simulink model "adarbha_HW9_sim"  (Simulink 7.7)
settings: Solver=ode1  StartTime=0.0  StopTime=900  FixedStep=0.01  RelTol=1e-2
undefined symbols (not defined in the file): area_sq_m, Cd, density, FUEL_FLOW, OMEGA_ICE, Q, R_batt, radius_wheel_m, rpm, Time, time_s, torque, TORQUE_ICE, V_o, vel_m_s, Velocity_kph, weight_N
libraries: simulink x6
settings Model: Creator=Arjun  LastModifiedBy=Arjun

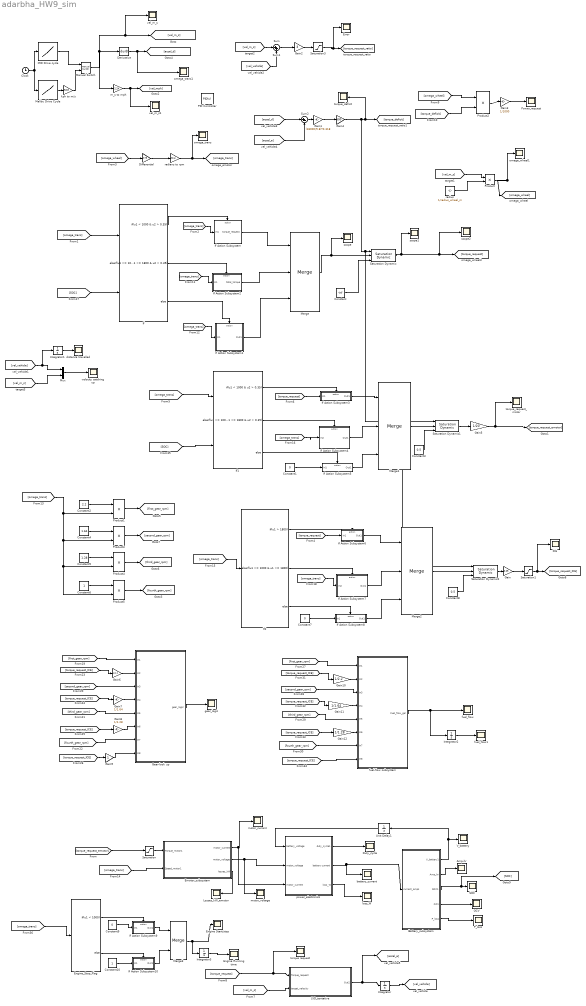
== system adarbha_HW9_sim ==
  Amp-hr : Scope
      settings: SaveName=ScopeData32
  Battery_subsystem : Subsystem
  Clock : Clock
      settings: Decimation=10
  Constant : Constant  Value=-Inf
  Constant1 : Constant  Value=0
  Constant10 : Constant
  Constant2 : Constant  Value=2.2
  Constant3 : Constant  Value=0.5
  Constant4 : Constant  Value=1.64
  Constant5 : Constant  Value=1.28
  Constant6 : Constant
  Constant7 : Constant  Value=0
  Constant8 : Constant  Value=0.5
  Constant9 : Constant  Value=0
  Derivative : Derivative
  Differential : Gain  Gain=3.73
  Duty_cycle : Scope
      settings: SaveName=ScopeData34
  Emotor_subsystem : Subsystem
  Engine Running time : Scope
      settings: SaveName=ScopeData61
  Engine Start/stop : Scope
      settings: SaveName=ScopeData60
  Engine_Stop_Flag : If  IfExpression=u1 < 1000
  Error : Scope
      settings: SaveName=ScopeData17
  Gain : Gain  Gain=0.25
  Gain1 : Gain  Gain=(18000/9.8)*0.318
  Gain10 : Gain  Gain=1/2.2
  Gain11 : Gain  Gain=1/1.64
  Gain12 : Gain  Gain=1/1.28
  Gain2 : Gain  Gain=3
  Gain3 : Gain  Gain=1/1000
  Gain4 : Gain  Gain=500
  Gain5 : Gain  Gain=1/20
  Gain6 : Gain  Gain=1/2.2
  Gain7 : Gain  Gain=1/1.64
  Gain8 : Gain  Gain=1/1.28
  Gain9 : Gain
  Gear-look up : Subsystem
  ICE : Scope
      settings: SaveName=ScopeData44
  If : If  NumInputs=2  IfExpression=u1 < 1000 & u2 > 0.35  ElseIfExpressions=u1 >= 1000 | u1 <= 1800 & u2 > 0.35
  If Action Subsystem : Subsystem  TreatAsAtomicUnit=on
  If Action Subsystem1 : Subsystem  TreatAsAtomicUnit=on
  If Action Subsystem10 : Subsystem  TreatAsAtomicUnit=on
  If Action Subsystem2 : Subsystem  TreatAsAtomicUnit=on
  If Action Subsystem3 : Subsystem  TreatAsAtomicUnit=on
  If Action Subsystem4 : Subsystem  TreatAsAtomicUnit=on
  If Action Subsystem5 : Subsystem  TreatAsAtomicUnit=on
  If Action Subsystem6 : Subsystem  TreatAsAtomicUnit=on
  If Action Subsystem7 : Subsystem  TreatAsAtomicUnit=on
  If Action Subsystem8 : Subsystem  TreatAsAtomicUnit=on
  If Action Subsystem9 : Subsystem  TreatAsAtomicUnit=on
  If1 : If  NumInputs=2  IfExpression=u1 < 1000 & u2 > 0.35  ElseIfExpressions=u1 >= 1000 | u1 <= 1800 & u2 > 0.35
  If2 : If  IfExpression=u1 > 1800  ElseIfExpressions=u1 >= 1000 & u1 <= 1800
  Integrator{,1..3} (4 alike) : Integrator
  LVD_tentative : Subsystem
  Losses_kW_emotor : Scope
      settings: SaveName=ScopeData36
  MID Drive cycle : Lookup_n-D  NumberOfTableDimensions=1  BreakpointsForDimension1=time_s  Table=vel_m_s  RndMeth=Simplest  InputSameDT=on
  Malibu Drive Cycle : Lookup_n-D  NumberOfTableDimensions=1  BreakpointsForDimension1=Time  Table=Velocity_kph  RndMeth=Simplest  InputSameDT=on
  Manual Switch : simulink/Signal Routing/Manual Switch  SystemSampleTime=-1  sw=0  action=0  varsize=off
  Merge : Merge  Inputs=3
  Merge1 : Merge  Inputs=3
  Merge2 : Merge  Inputs=3
  Merge3 : Merge
  Mux : Mux  Inputs=2
  OCV : Scope
      settings: SaveName=ScopeData31
  PID Controller : simulink/Continuous/PID Controller  SystemSampleTime=-1  Controller=PID  TimeDomain=Continuous-time  SampleTime=1  IntegratorMethod=Forward Euler  FilterMethod=Forward Euler  Form=Parallel  P=0.3  I=0  D=0.5  N=100  InitialConditionSource=internal  InitialConditionForIntegrator=0  InitialConditionForFilter=0  ExternalReset=none  LimitOutput=off  UpperSaturationLimit=inf  LowerSaturationLimit=-inf  LinearizeAsGain=off  AntiWindupMode=none  Kb=1  TrackingMode=off  Kt=1  PParamMin=[]  PParamMax=[]  IParamMin=[]  IParamMax=[]  DParamMin=[]  DParamMax=[]  NParamMin=[]  NParamMax=[]  KbParamMin=[]  KbParamMax=[]  KtParamMin=[]  KtParamMax=[]  POutMin=[]  POutMax=[]  IOutMin=[]  IOutMax=[]  DOutMin=[]  DOutMax=[]  NOutMin=[]  NOutMax=[]  KbOutMin=[]  KbOutMax=[]  KtOutMin=[]  KtOutMax=[]  IntegratorOutMin=[]  IntegratorOutMax=[]  FilterOutMin=[]  FilterOutMax=[]  SumOutMin=[]  SumOutMax=[]  SumI1OutMin=[]  SumI1OutMax=[]  SumI2OutMin=[]  SumI2OutMax=[]  SumI3OutMin=[]  SumI3OutMax=[]  SumDOutMin=[]  SumDOutMax=[]  SaturationOutMin=[]  SaturationOutMax=[]  IntegratorContinuousStateAttributes=''  IntegratorStateMustResolveToSignalObject=off  IntegratorRTWStateStorageClass=Auto  FilterContinuousStateAttributes=''  FilterStateMustResolveToSignalObject=off  FilterRTWStateStorageClass=Auto
  P_loss : Scope
      settings: SaveName=ScopeData33
  Power_request : Scope
      settings: SaveName=ScopeData19
  Product{,1..5} (6 alike) : Product  RndMeth=Zero
  SOC : Scope
      settings: SaveName=ScopeData37
  Saturation : Saturate  UpperLimit=100000000  LowerLimit=-2160
  Saturation Dynamic : simulink/Discontinuities/Saturation Dynamic  SystemSampleTime=-1  OutMin=1  OutMax=[]  OutDataTypeStr=Inherit: Same as second input  OutDataType=fixdt(1, 16)  OutScaling=2^-10  DoSatur=off
  Saturation Dynamic1 : simulink/Discontinuities/Saturation Dynamic  SystemSampleTime=-1  OutMin=1  OutMax=[]  OutDataTypeStr=Inherit: Same as second input  OutDataType=fixdt(1, 16)  OutScaling=2^-10  DoSatur=off
  Saturation Dynamic2 : simulink/Discontinuities/Saturation Dynamic  SystemSampleTime=-1  OutMin=1  OutMax=[]  OutDataTypeStr=Inherit: Same as second input  OutDataType=fixdt(1, 16)  OutScaling=2^-10  DoSatur=off
  Saturation1 : Saturate  UpperLimit=10000000  LowerLimit=0
  Saturation3 : Saturate  UpperLimit=1  LowerLimit=-1
  Sum : Sum  Inputs=|+-
  Sum1 : Sum  Inputs=|++
  Sum2 : Sum  Inputs=|+-
  Unit Delay1 : UnitDelay  SampleTime=-1
  V_battery : Scope
      settings: TimeRange=500  YMin=-50  YMax=300  SaveName=ScopeData29
  battery_current : Scope
      settings: SaveName=ScopeData24
  distance travelled : Scope
      settings: SaveName=ScopeData25
  fuel-flow subsystem : Subsystem
  fuel_flow : Scope
      settings: SaveName=ScopeData46
  fuel_flow1 : Scope
      settings: SaveName=ScopeData59
  gear_logic : Scope
      settings: SaveName=ScopeData45
  kph to m/s : Gain  Gain=5/18
  loss_W : Scope
      settings: SaveName=ScopeData38
  m_s to mph : Gain  Gain=2.24
  motor_current : Scope
      settings: SaveName=ScopeData39
  motor_voltage : Scope
      settings: SaveName=ScopeData26
  omega_trans : Scope
      settings: YMin=0  YMax=40  SaveName=ScopeData16
  omega_trans1 : Scope
      settings: YMin=0  YMax=40  SaveName=ScopeData41
  omega_wheel1 : Scope
      settings: SaveName=ScopeData4
  power_electronics : Subsystem
  radians to rpm : Gain  Gain=30/pi
  radius : Constant  Value=1/radius_wheel_m
  scope : Scope
      settings: SaveName=ScopeData3
  scope1 : Scope
      settings: SaveName=ScopeData7
  scope2 : Scope
      settings: SaveName=ScopeData20
  torque request : Scope
      settings: SaveName=ScopeData12
  torque_deficit : Scope
  torque_request_motor : Scope
  vel_m_s : Scope
      settings: TimeRange=49.80784012298233  YMin=0  YMax=30  SaveName=ScopeData21
  vel_m_s1 : Scope
      settings: YMin=0  YMax=40  SaveName=ScopeData28
  velocity catching up : Scope
      settings: TimeRange=765.8724058416602  YMin=-1e+049  YMax=9.000000000000001e+049  SaveName=ScopeData18  SampleTime=800
  wires:
  m_s to mph/1 -> [vel_mph], vel_m_s1/1
  Clock/1 -> MID Drive cycle/1, Malibu Drive Cycle/1
  [vel_m_s] -> Product/1
  Product/1 -> [omega_wheel], omega_wheel1/1
  radius/1 -> Product/2
  [omega_wheel] -> Differential/1
  [vel_m_s] -> LVD_tentative/2(target_velocity)
  [torque_request] -> LVD_tentative/1(Torque_request), torque request/1
  Integrator/1 -> [vel_vehicle]
  LVD_tentative/1(Out2) -> Integrator/1, [accel_a]
  [vel_m_s] -> Sum/1
  [vel_vehicle] -> Sum/2
  [vel_m_s] -> Mux/2
  [vel_vehicle] -> Mux/1, Integrator1/1
  MID Drive cycle/1 -> Manual Switch/1
  Manual Switch/1 -> m_s to mph/1, [vel_m_s], vel_m_s/1, Derivative/1
  Malibu Drive Cycle/1 -> kph to m/s/1
  kph to m/s/1 -> Manual Switch/2
  Integrator1/1 -> distance travelled/1
  Gain2/1 -> Saturation3/1
  Sum/1 -> Gain2/1
  Mux/1 -> velocity catching up/1
  Derivative/1 -> [accel_d], omega_trans1/1
  [accel_d] -> Sum2/1
  [accel_a] -> Sum2/2
  Sum2/1 -> Gain1/1
  Gain1/1 -> Gain4/1
  Saturation3/1 -> [torque_request_ratio], Error/1
  [omega_trans] -> If/1
  If/1 -> If Action Subsystem/Action
  [omega_trans] -> If Action Subsystem/1(In1)
  If/2 -> If Action Subsystem2/Action
  [omega_wheel] -> Product2/1
  [torque_deficit] -> Product2/2
  Product2/1 -> Gain3/1
  Gain3/1 -> Power_request/1
  [omega_trans] -> If Action Subsystem2/1(In1)
  radians to rpm/1 -> [omega_trans], omega_trans/1
  Differential/1 -> radians to rpm/1
  [omega_trans] -> If Action Subsystem1/1(In1)
  If/3 -> If Action Subsystem1/Action
  If Action Subsystem/1(torque_request) -> Merge/1
  If Action Subsystem2/1(total_torque) -> Merge/2
  If Action Subsystem1/1(Out1) -> Merge/3
  Saturation Dynamic/1 -> scope1/1, [torque_request], scope2/1
  Constant/1 -> Saturation Dynamic/3
  Merge/1 -> Saturation Dynamic/2, scope/1
  [omega_trans] -> If1/1
  If1/1 -> If Action Subsystem3/Action
  [torque_request] -> If Action Subsystem3/1(In1)
  If1/2 -> If Action Subsystem4/Action
  If1/3 -> If Action Subsystem5/Action
  Constant1/1 -> If Action Subsystem5/1(In1)
  If Action Subsystem3/1(Out1) -> Merge1/1
  If Action Subsystem4/1(Out1) -> Merge1/2
  If Action Subsystem5/1(Out1) -> Merge1/3
  power_electronics/2(battery current) -> battery_current/1, Battery_subsystem/1(current_amps)
  Battery_subsystem/1(V_battery1) -> V_battery/1, Unit Delay1/1
  Battery_subsystem/3(SOC1) -> SOC/1, [SOC]
  power_electronics/3(loss_W) -> loss_W/1
  power_electronics/1(duty_cycle1) -> Duty_cycle/1
  Battery_subsystem/2(Amp_hr) -> Amp-hr/1
  Battery_subsystem/4(OCV) -> OCV/1
  Battery_subsystem/5(P_loss) -> P_loss/1
  Unit Delay1/1 -> power_electronics/1(battery_voltage)
  Emotor_subsystem/3(losses_kW) -> Losses_kW_emotor/1
  Emotor_subsystem/2(motor_voltage) -> power_electronics/2(motor_voltage), motor_voltage/1
  Emotor_subsystem/1(motor_current) -> motor_current/1, power_electronics/3(motor_current)
  [torque_request_emotor] -> Saturation/1
  [omega_trans] -> Emotor_subsystem/2(Speed_motor1)
  Gain4/1 -> [torque_deficit], torque_deficit/1, Saturation Dynamic/1, Saturation Dynamic1/1, Saturation Dynamic2/1
  [omega_trans] -> If Action Subsystem4/1(In2)
  Merge1/1 -> Saturation Dynamic1/2
  Constant3/1 -> Saturation Dynamic1/3
  Saturation Dynamic1/1 -> Gain5/1
  Saturation/1 -> Emotor_subsystem/1(Torque_motor1)
  [omega_trans] -> Product1/2, Product3/2, Product4/2, Product5/2
  Constant2/1 -> Product1/1
  Constant4/1 -> Product3/1
  Constant5/1 -> Product4/1
  Constant6/1 -> Product5/1
  Product1/1 -> [first_gear_rpm]
  Product3/1 -> [second_gear_rpm]
  Product4/1 -> [third_gear_rpm]
  Product5/1 -> [fourth_gear_rpm]
  [omega_trans] -> If2/1
  If2/1 -> If Action Subsystem6/Action
  If2/2 -> If Action Subsystem7/Action
  [omega_trans] -> If Action Subsystem7/1(In2)
  If2/3 -> If Action Subsystem8/Action
  Constant7/1 -> If Action Subsystem8/1(In1)
  If Action Subsystem8/1(Out1) -> Merge2/3
  If Action Subsystem7/1(Out1) -> Merge2/2
  If Action Subsystem6/1(Out1) -> Merge2/1
  Merge2/1 -> Saturation Dynamic2/2
  Constant8/1 -> Saturation Dynamic2/3
  Saturation Dynamic2/1 -> Gain/1
  Gain/1 -> Saturation1/1
  Saturation1/1 -> [torque_request_ICE], ICE/1
  [first_gear_rpm] -> Gear-look up/1(In1)
  [torque_request_ICE] -> Gain6/1
  [second_gear_rpm] -> Gear-look up/3(In3)
  [torque_request_ICE] -> Gain7/1
  [third_gear_rpm] -> Gear-look up/5(In5)
  [fourth_gear_rpm] -> Gear-look up/7(In7)
  Gear-look up/1(gear_logic) -> gear_logic/1
  Gain5/1 -> [torque_request_emotor], torque_request_motor/1
  [torque_request_ICE] -> Gain8/1
  [torque_request_ICE] -> Gain9/1
  [first_gear_rpm] -> fuel-flow subsystem/1(In1)
  [torque_request_ICE] -> Gain10/1
  [second_gear_rpm] -> fuel-flow subsystem/3(In3)
  [torque_request_ICE] -> Gain11/1
  [third_gear_rpm] -> fuel-flow subsystem/5(In5)
  [fourth_gear_rpm] -> fuel-flow subsystem/7(In7)
  [torque_request_ICE] -> Gain12/1
  [torque_request_ICE] -> fuel-flow subsystem/8(In8)
  fuel-flow subsystem/1(Fuel_flow_gal) -> fuel_flow/1, Integrator2/1
  Integrator2/1 -> fuel_flow1/1
  [torque_request] -> If Action Subsystem6/1(In1)
  [SOC] -> If/2
  [SOC] -> If1/2
  [omega_trans] -> Engine_Stop_Flag/1
  Engine_Stop_Flag/1 -> If Action Subsystem9/Action
  Constant9/1 -> If Action Subsystem9/1(In1)
  Engine_Stop_Flag/2 -> If Action Subsystem10/Action
  Constant10/1 -> If Action Subsystem10/1(In1)
  If Action Subsystem9/1(Out1) -> Merge3/1
  If Action Subsystem10/1(Out1) -> Merge3/2
  Merge3/1 -> Engine Start/stop/1, Integrator3/1
  Gain6/1 -> Gear-look up/2(In2)
  Gain7/1 -> Gear-look up/4(In4)
  Gain8/1 -> Gear-look up/6(In6)
  Gain9/1 -> Gear-look up/8(In8)
  Gain10/1 -> fuel-flow subsystem/2(In2)
  Gain11/1 -> fuel-flow subsystem/4(In4)
  Gain12/1 -> fuel-flow subsystem/6(In6)
  Integrator3/1 -> Engine Running time/1

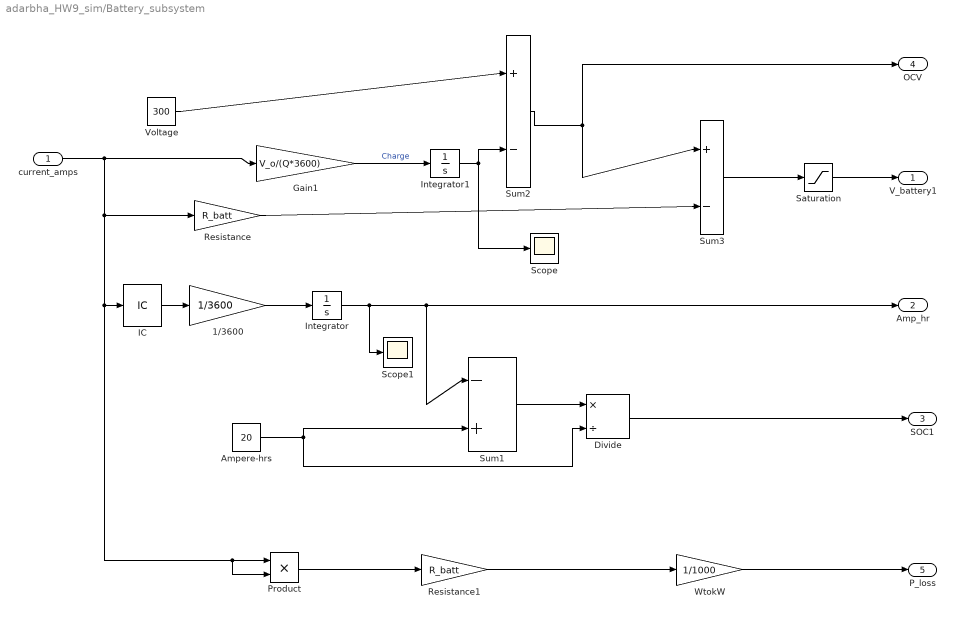
== system adarbha_HW9_sim/Battery_subsystem ==
  current_amps : Inport
  1/3600 : Gain  Gain=1/3600
  Ampere-hrs : Constant  Value=20
  Divide : Product  Inputs=*/
  Gain1 : Gain  Gain=V_o/(Q*3600)
  IC : InitialCondition  Value=0.1
  Integrator : Integrator  InitialCondition=0.1  LimitOutput=on  UpperSaturationLimit=20  LowerSaturationLimit=0
  Integrator1 : Integrator  LimitOutput=on  UpperSaturationLimit=300  LowerSaturationLimit=0
  Product : Product  RndMeth=Zero
  Resistance : Gain  Gain=R_batt
  Resistance1 : Gain  Gain=R_batt
  Saturation : Saturate  UpperLimit=300  LowerLimit=1  ZeroCross=off
  Scope : Scope
  Scope1 : Scope
      settings: SaveName=ScopeData3
  Sum1 : Sum  Inputs=|-+
  Sum2 : Sum  Inputs=|+-
  Sum3 : Sum  Inputs=|+-
  Voltage : Constant  Value=300
  WtokW : Gain  Gain=1/1000
  V_battery1 : Outport
  Amp_hr : Outport  Port=2
  SOC1 : Outport  Port=3
  OCV : Outport  Port=4
  P_loss : Outport  Port=5
  wires:
  Gain1/1 -> Integrator1/1  "Charge"
  Integrator1/1 -> Sum2/2, Scope/1
  Resistance/1 -> Sum3/2
  Ampere-hrs/1 -> Sum1/2, Divide/2
  Sum1/1 -> Divide/1
  Divide/1 -> SOC1/1
  current_amps/1 -> Gain1/1, Product/1, Product/2, IC/1, Resistance/1
  Product/1 -> Resistance1/1
  Resistance1/1 -> WtokW/1
  1/3600/1 -> Integrator/1
  Integrator/1 -> Amp_hr/1, Sum1/1, Scope1/1
  Sum3/1 -> Saturation/1
  Voltage/1 -> Sum2/1
  Sum2/1 -> Sum3/1, OCV/1
  Saturation/1 -> V_battery1/1
  WtokW/1 -> P_loss/1
  IC/1 -> 1/3600/1

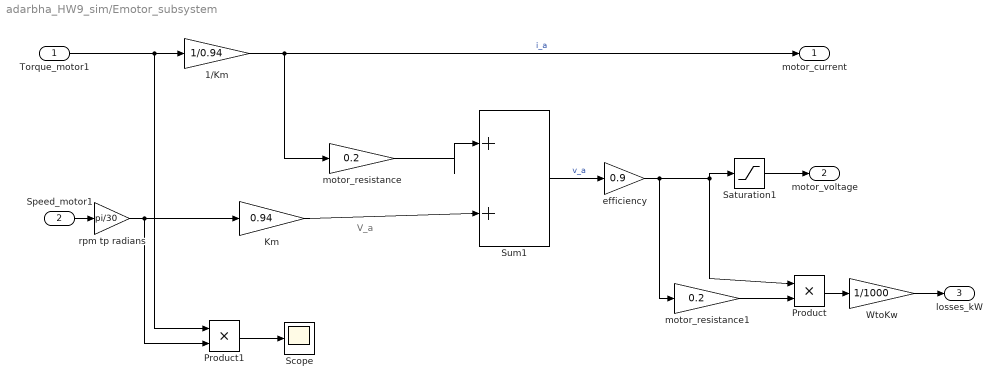
== system adarbha_HW9_sim/Emotor_subsystem ==
  note: V_a
  Torque_motor1 : Inport
  Speed_motor1 : Inport  Port=2
  1/Km : Gain  Gain=1/0.94
  Km : Gain  Gain=0.94
  Product : Product  RndMeth=Zero
  Product1 : Product  RndMeth=Zero
  Saturation1 : Saturate  UpperLimit=300  LowerLimit=0
  Scope : Scope
      settings: SaveName=ScopeData30
  Sum1 : Sum  Inputs=|++
  WtoKw : Gain  Gain=1/1000
  efficiency : Gain  Gain=0.9
  motor_resistance : Gain  Gain=0.2
  motor_resistance1 : Gain  Gain=0.2
  rpm tp radians : Gain  Gain=pi/30
  motor_current : Outport
  motor_voltage : Outport  Port=2
  losses_kW : Outport  Port=3
  wires:
  Torque_motor1/1 -> 1/Km/1, Product1/1
  Speed_motor1/1 -> rpm tp radians/1
  Km/1 -> Sum1/2
  1/Km/1 -> motor_resistance/1, motor_current/1  "i_a"
  motor_resistance/1 -> Sum1/1
  motor_resistance1/1 -> Product/2
  Product/1 -> WtoKw/1
  WtoKw/1 -> losses_kW/1
  Saturation1/1 -> motor_voltage/1
  Product1/1 -> Scope/1
  efficiency/1 -> motor_resistance1/1, Product/1, Saturation1/1
  Sum1/1 -> efficiency/1  "v_a"
  rpm tp radians/1 -> Km/1, Product1/2

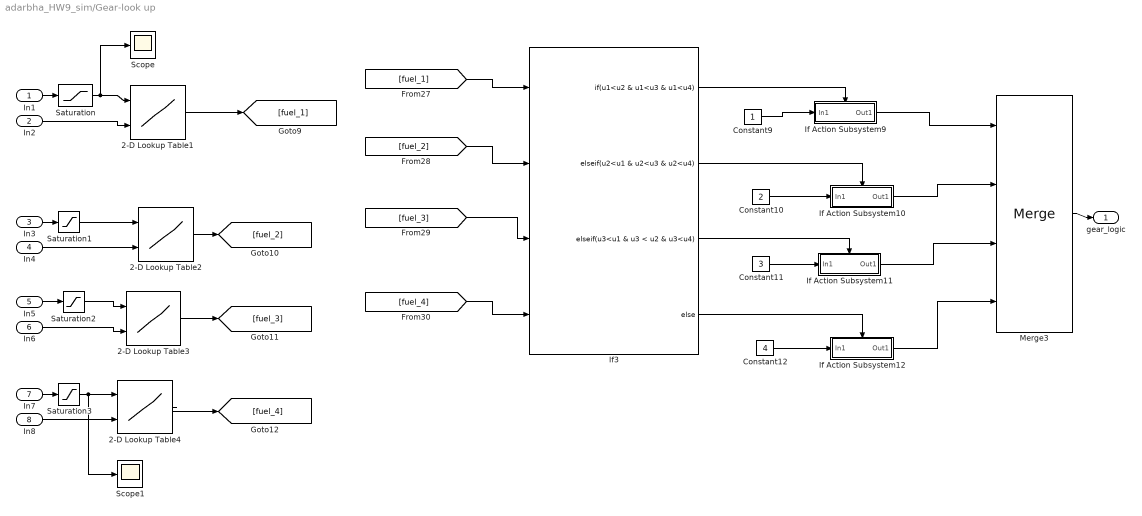
== system adarbha_HW9_sim/Gear-look up ==
  In1 : Inport
  In2 : Inport  Port=2
  In3 : Inport  Port=3
  In4 : Inport  Port=4
  In5 : Inport  Port=5
  In6 : Inport  Port=6
  In7 : Inport  Port=7
  In8 : Inport  Port=8
  2-D Lookup Table{1..4} (4 alike) : Lookup_n-D  BreakpointsForDimension1=OMEGA_ICE  BreakpointsForDimension2=TORQUE_ICE  Table=FUEL_FLOW  RndMeth=Simplest  InputSameDT=on
  Constant10 : Constant  Value=2
  Constant11 : Constant  Value=3
  Constant12 : Constant  Value=4
  Constant9 : Constant
  If Action Subsystem10 : Subsystem  TreatAsAtomicUnit=on
  If Action Subsystem11 : Subsystem  TreatAsAtomicUnit=on
  If Action Subsystem12 : Subsystem  TreatAsAtomicUnit=on
  If Action Subsystem9 : Subsystem  TreatAsAtomicUnit=on
  If3 : If  NumInputs=4  IfExpression=u1<u2 & u1<u3 & u1<u4  ElseIfExpressions=u2<u1 & u2<u3 & u2<u4, u3<u1 & u3 < u2 & u3<u4
  Merge3 : Merge  Inputs=4
  Saturation{,1..3} (4 alike) : Saturate  UpperLimit=Inf  LowerLimit=1000
  Scope : Scope
      settings: SaveName=ScopeData53
  Scope1 : Scope
      settings: SaveName=ScopeData54
  gear_logic : Outport
  wires:
  2-D Lookup Table1/1 -> [fuel_1]
  2-D Lookup Table2/1 -> [fuel_2]
  2-D Lookup Table3/1 -> [fuel_3]
  2-D Lookup Table4/1 -> [fuel_4]
  [fuel_1] -> If3/1
  [fuel_2] -> If3/2
  [fuel_3] -> If3/3
  [fuel_4] -> If3/4
  If3/1 -> If Action Subsystem9/Action
  Constant9/1 -> If Action Subsystem9/1(In1)
  If3/2 -> If Action Subsystem10/Action
  Constant10/1 -> If Action Subsystem10/1(In1)
  Constant11/1 -> If Action Subsystem11/1(In1)
  Constant12/1 -> If Action Subsystem12/1(In1)
  If3/4 -> If Action Subsystem12/Action
  If3/3 -> If Action Subsystem11/Action
  If Action Subsystem9/1(Out1) -> Merge3/1
  If Action Subsystem10/1(Out1) -> Merge3/2
  If Action Subsystem11/1(Out1) -> Merge3/3
  If Action Subsystem12/1(Out1) -> Merge3/4
  In1/1 -> Saturation/1
  In2/1 -> 2-D Lookup Table1/2
  In3/1 -> Saturation1/1
  In4/1 -> 2-D Lookup Table2/2
  In5/1 -> Saturation2/1
  Merge3/1 -> gear_logic/1
  In6/1 -> 2-D Lookup Table3/2
  In7/1 -> Saturation3/1
  In8/1 -> 2-D Lookup Table4/2
  Saturation/1 -> 2-D Lookup Table1/1, Scope/1
  Saturation1/1 -> 2-D Lookup Table2/1
  Saturation2/1 -> 2-D Lookup Table3/1
  Saturation3/1 -> 2-D Lookup Table4/1, Scope1/1

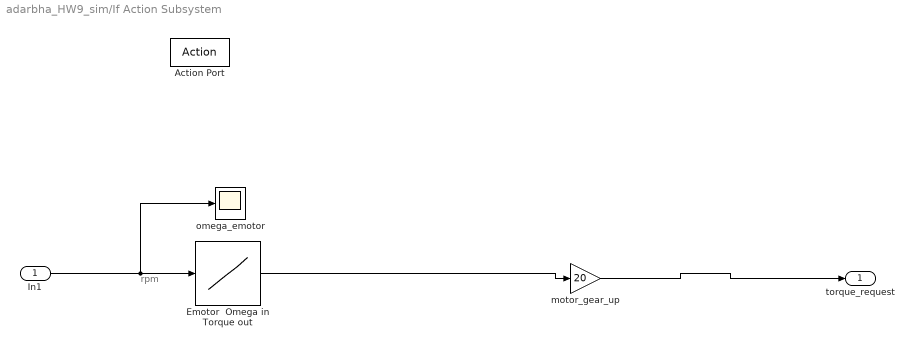
== system adarbha_HW9_sim/If Action Subsystem ==
  note: rpm
  In1 : Inport
  Action Port : ActionPort  ActionType=then
  Emotor  Omega in Torque out : Lookup_n-D  NumberOfTableDimensions=1  BreakpointsForDimension1=rpm  Table=torque  RndMeth=Simplest  InputSameDT=on
  motor_gear_up : Gain  Gain=20
  omega_emotor : Scope
      settings: SaveName=ScopeData2
  torque_request : Outport
  wires:
  In1/1 -> Emotor  Omega in Torque out/1, omega_emotor/1
  Emotor  Omega in Torque out/1 -> motor_gear_up/1
  motor_gear_up/1 -> torque_request/1

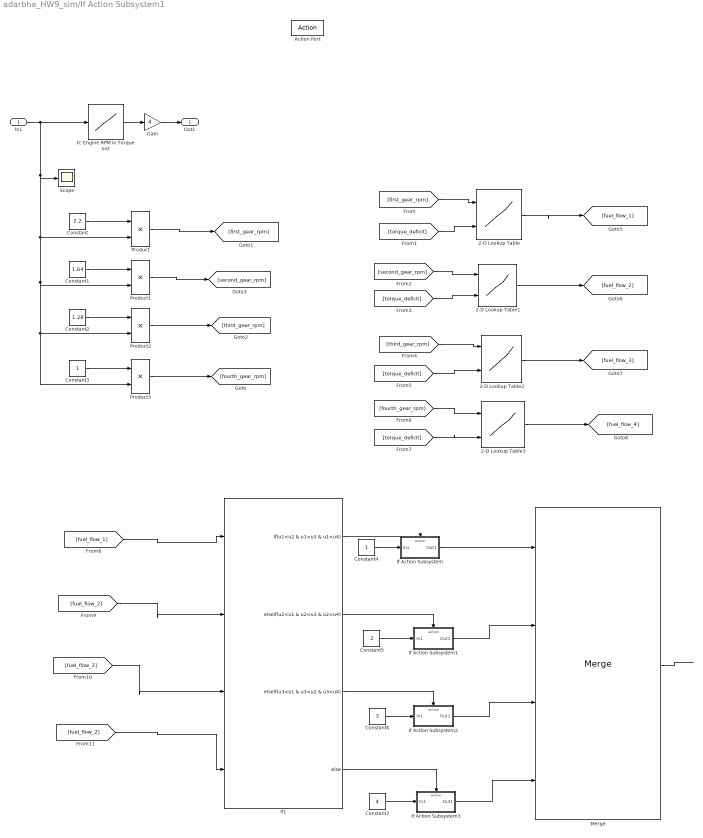
== system adarbha_HW9_sim/If Action Subsystem1 ==
  In1 : Inport
  Action Port : ActionPort  ActionType=else
  2-D Lookup Table{,1..3} (4 alike) : Lookup_n-D  BreakpointsForDimension1=OMEGA_ICE  BreakpointsForDimension2=TORQUE_ICE  Table=FUEL_FLOW  RndMeth=Simplest  InputSameDT=on
  Constant : Constant  Value=2.2
  Constant1 : Constant  Value=1.64
  Constant2 : Constant  Value=1.28
  Constant3 : Constant
  Constant4 : Constant
  Constant5 : Constant  Value=2
  Constant6 : Constant  Value=3
  Constant7 : Constant  Value=4
  Gain : Gain  Gain=4
  IC Engine RPM in Torque out : Lookup_n-D  NumberOfTableDimensions=1  BreakpointsForDimension1=TORQUE_ICE  Table=OMEGA_ICE  RndMeth=Simplest  InputSameDT=on
  If Action Subsystem : Subsystem  TreatAsAtomicUnit=on
  If Action Subsystem1 : Subsystem  TreatAsAtomicUnit=on
  If Action Subsystem2 : Subsystem  TreatAsAtomicUnit=on
  If Action Subsystem3 : Subsystem  TreatAsAtomicUnit=on
  If1 : If  NumInputs=4  IfExpression=u1<u2 & u1<u3 & u1<u4  ElseIfExpressions=u2<u1 & u2<u3 & u2<u4, u3<u1 & u3<u2 & u3<u4
  Merge : Merge  Inputs=4
  Product{,1..3} (4 alike) : Product  RndMeth=Zero
  Scope : Scope
      settings: SaveName=ScopeData40
  Out1 : Outport
  wires:
  In1/1 -> IC Engine RPM in Torque out/1, Product/2, Product1/2, Product2/2, Product3/2, Scope/1
  IC Engine RPM in Torque out/1 -> Gain/1
  Gain/1 -> Out1/1
  Constant/1 -> Product/1
  Constant1/1 -> Product1/1
  Constant2/1 -> Product2/1
  Constant3/1 -> Product3/1
  Product/1 -> [first_gear_rpm]
  Product1/1 -> [second_gear_rpm]
  Product2/1 -> [third_gear_rpm]
  Product3/1 -> [fourth_gear_rpm]
  [first_gear_rpm] -> 2-D Lookup Table/1
  [torque_deficit] -> 2-D Lookup Table/2
  [second_gear_rpm] -> 2-D Lookup Table1/1
  [torque_deficit] -> 2-D Lookup Table1/2
  [third_gear_rpm] -> 2-D Lookup Table2/1
  [torque_deficit] -> 2-D Lookup Table2/2
  [fourth_gear_rpm] -> 2-D Lookup Table3/1
  [torque_deficit] -> 2-D Lookup Table3/2
  2-D Lookup Table/1 -> [fuel_flow_1]
  2-D Lookup Table1/1 -> [fuel_flow_2]
  2-D Lookup Table2/1 -> [fuel_flow_3]
  2-D Lookup Table3/1 -> [fuel_flow_4]
  [fuel_flow_1] -> If1/1
  [fuel_flow_2] -> If1/2
  [fuel_flow_2] -> If1/3
  [fuel_flow_2] -> If1/4
  If1/1 -> If Action Subsystem/Action
  Constant4/1 -> If Action Subsystem/1(In1)
  If1/2 -> If Action Subsystem1/Action
  If1/3 -> If Action Subsystem2/Action
  If1/4 -> If Action Subsystem3/Action
  Constant5/1 -> If Action Subsystem1/1(In1)
  Constant6/1 -> If Action Subsystem2/1(In1)
  Constant7/1 -> If Action Subsystem3/1(In1)
  If Action Subsystem/1(Out1) -> Merge/1
  If Action Subsystem1/1(Out1) -> Merge/2
  If Action Subsystem2/1(Out1) -> Merge/3
  If Action Subsystem3/1(Out1) -> Merge/4
  Merge/1 -> ?

== system adarbha_HW9_sim/If Action Subsystem10 ==
  In1 : Inport
  Action Port : ActionPort  ActionType=else
  Out1 : Outport
  wires:
  In1/1 -> Out1/1

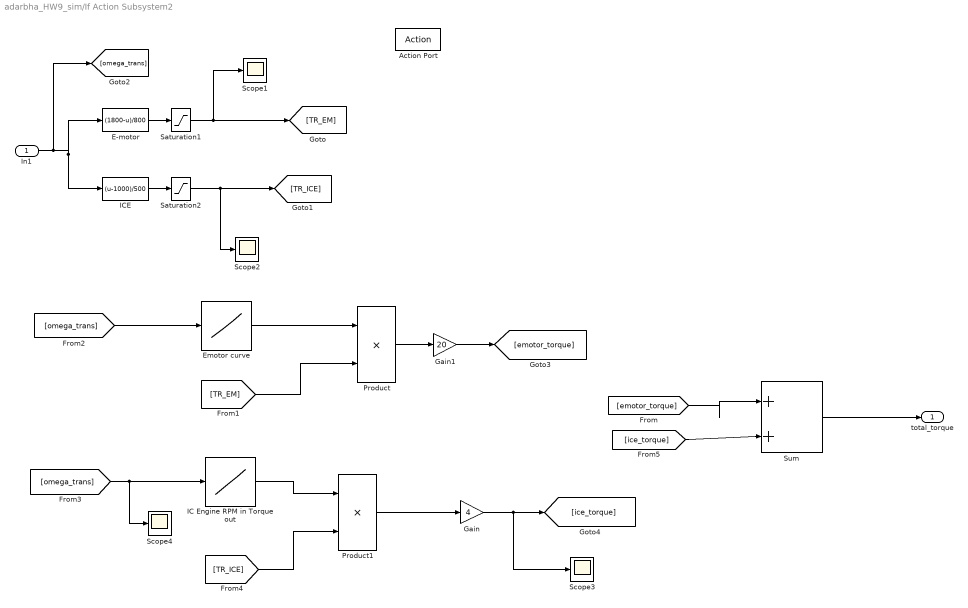
== system adarbha_HW9_sim/If Action Subsystem2 ==
  In1 : Inport
  Action Port : ActionPort  ActionType=elseif
  E-motor : Fcn  Expr=(1800-u)/800
  Emotor curve : Lookup_n-D  NumberOfTableDimensions=1  BreakpointsForDimension1=rpm  Table=torque  RndMeth=Simplest  InputSameDT=on
  Gain : Gain  Gain=4
  Gain1 : Gain  Gain=20
  IC Engine RPM in Torque out : Lookup_n-D  NumberOfTableDimensions=1  BreakpointsForDimension1=TORQUE_ICE  Table=OMEGA_ICE  RndMeth=Simplest  InputSameDT=on
  ICE : Fcn  Expr=(u-1000)/500
  Product : Product  RndMeth=Zero
  Product1 : Product  RndMeth=Zero
  Saturation1 : Saturate  UpperLimit=1  LowerLimit=0
  Saturation2 : Saturate  UpperLimit=1  LowerLimit=0
  Scope{1..4} (4 alike) : Scope
      Scope1 settings: SaveName=ScopeData22
      Scope2 settings: SaveName=ScopeData23
      Scope3 settings: SaveName=ScopeData48
      Scope4 settings: SaveName=ScopeData49
  Sum : Sum  Inputs=|++
  total_torque : Outport
  wires:
  In1/1 -> E-motor/1, ICE/1, [omega_trans]
  E-motor/1 -> Saturation1/1
  ICE/1 -> Saturation2/1
  Saturation1/1 -> [TR_EM], Scope1/1
  Saturation2/1 -> [TR_ICE], Scope2/1
  [omega_trans] -> Emotor curve/1
  Emotor curve/1 -> Product/1
  [TR_EM] -> Product/2
  Product/1 -> Gain1/1
  [omega_trans] -> IC Engine RPM in Torque out/1, Scope4/1
  IC Engine RPM in Torque out/1 -> Product1/1
  [TR_ICE] -> Product1/2
  Product1/1 -> Gain/1
  Sum/1 -> total_torque/1
  [ice_torque] -> Sum/2
  [emotor_torque] -> Sum/1
  Gain/1 -> [ice_torque], Scope3/1
  Gain1/1 -> [emotor_torque]

== system adarbha_HW9_sim/If Action Subsystem3 ==
  In1 : Inport
  Action Port : ActionPort  ActionType=then
  Out1 : Outport
  wires:
  In1/1 -> Out1/1

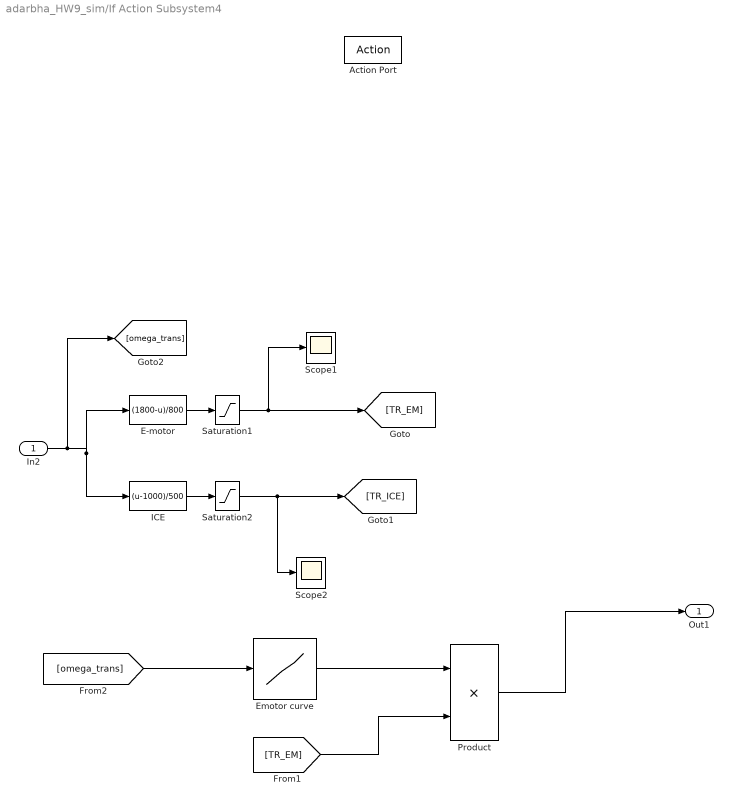
== system adarbha_HW9_sim/If Action Subsystem4 ==
  In2 : Inport
  Action Port : ActionPort  ActionType=elseif
  E-motor : Fcn  Expr=(1800-u)/800
  Emotor curve : Lookup_n-D  NumberOfTableDimensions=1  BreakpointsForDimension1=rpm  Table=torque  RndMeth=Simplest  InputSameDT=on
  ICE : Fcn  Expr=(u-1000)/500
  Product : Product  RndMeth=Zero
  Saturation1 : Saturate  UpperLimit=1  LowerLimit=0
  Saturation2 : Saturate  UpperLimit=1  LowerLimit=0
  Scope1 : Scope
      settings: SaveName=ScopeData11
  Scope2 : Scope
      settings: SaveName=ScopeData42
  Out1 : Outport
  wires:
  In2/1 -> E-motor/1, ICE/1, [omega_trans]
  E-motor/1 -> Saturation1/1
  ICE/1 -> Saturation2/1
  Saturation1/1 -> [TR_EM], Scope1/1
  Saturation2/1 -> [TR_ICE], Scope2/1
  [omega_trans] -> Emotor curve/1
  Emotor curve/1 -> Product/1
  [TR_EM] -> Product/2
  Product/1 -> Out1/1

== system adarbha_HW9_sim/If Action Subsystem5 ==
  In1 : Inport
  Action Port : ActionPort  ActionType=else
  Out1 : Outport
  wires:
  In1/1 -> Out1/1

== system adarbha_HW9_sim/If Action Subsystem6 ==
  In1 : Inport
  Action Port : ActionPort  ActionType=then
  Out1 : Outport
  wires:
  In1/1 -> Out1/1

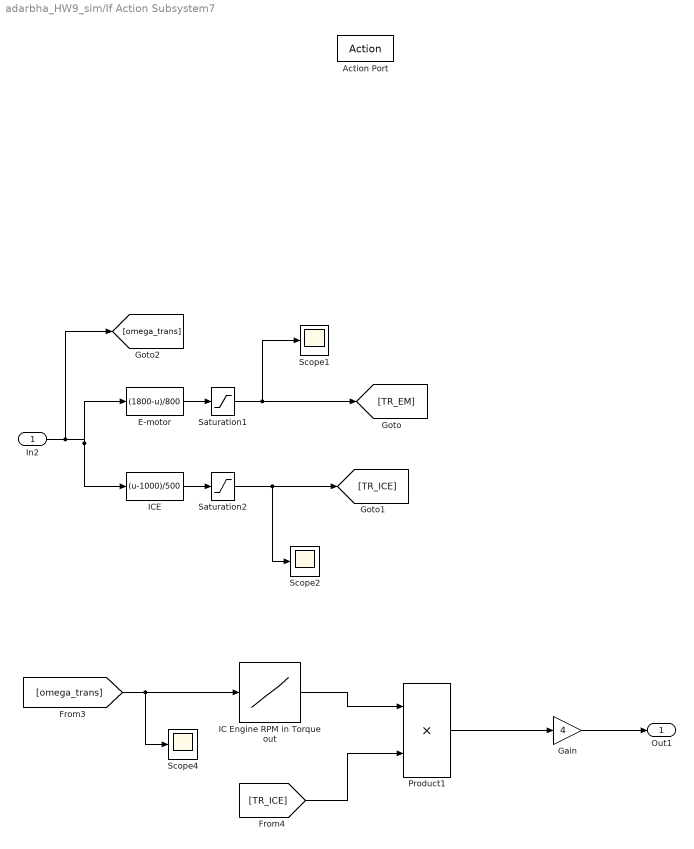
== system adarbha_HW9_sim/If Action Subsystem7 ==
  In2 : Inport
  Action Port : ActionPort  ActionType=elseif
  E-motor : Fcn  Expr=(1800-u)/800
  Gain : Gain  Gain=4
  IC Engine RPM in Torque out : Lookup_n-D  NumberOfTableDimensions=1  BreakpointsForDimension1=TORQUE_ICE  Table=OMEGA_ICE  RndMeth=Simplest  InputSameDT=on
  ICE : Fcn  Expr=(u-1000)/500
  Product1 : Product  RndMeth=Zero
  Saturation1 : Saturate  UpperLimit=1  LowerLimit=0
  Saturation2 : Saturate  UpperLimit=1  LowerLimit=0
  Scope1 : Scope
      settings: SaveName=ScopeData11
  Scope2 : Scope
      settings: SaveName=ScopeData42
  Scope4 : Scope
      settings: SaveName=ScopeData43
  Out1 : Outport
  wires:
  Saturation2/1 -> Scope2/1, [TR_ICE]
  Saturation1/1 -> Scope1/1, [TR_EM]
  ICE/1 -> Saturation2/1
  E-motor/1 -> Saturation1/1
  In2/1 -> [omega_trans], ICE/1, E-motor/1
  [omega_trans] -> IC Engine RPM in Torque out/1, Scope4/1
  IC Engine RPM in Torque out/1 -> Product1/1
  [TR_ICE] -> Product1/2
  Product1/1 -> Gain/1
  Gain/1 -> Out1/1

== system adarbha_HW9_sim/If Action Subsystem8 ==
  In1 : Inport
  Action Port : ActionPort  ActionType=else
  Out1 : Outport
  wires:
  In1/1 -> Out1/1

== system adarbha_HW9_sim/If Action Subsystem9 ==
  In1 : Inport
  Action Port : ActionPort  ActionType=then
  Out1 : Outport
  wires:
  In1/1 -> Out1/1

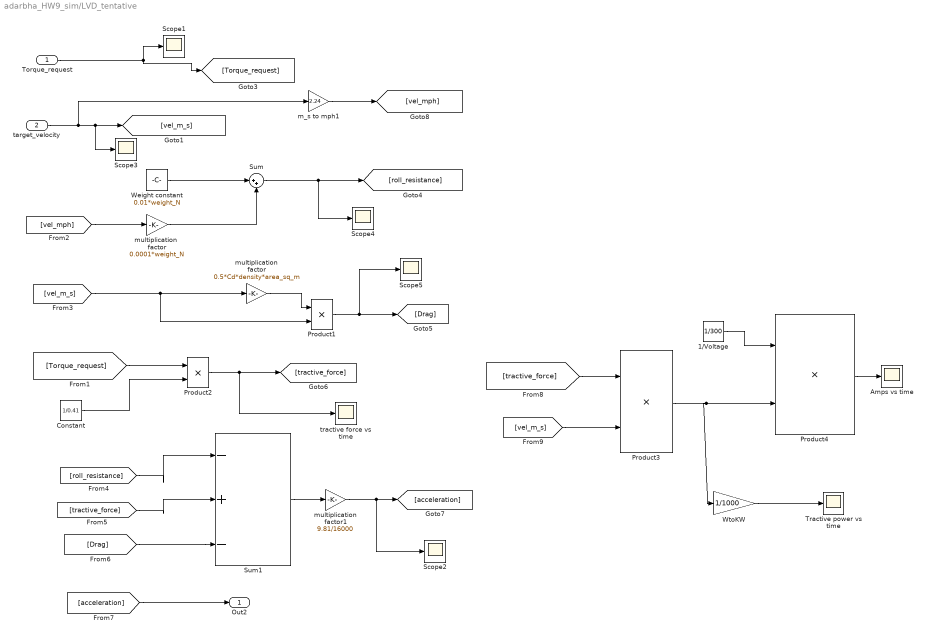
== system adarbha_HW9_sim/LVD_tentative ==
  Torque_request : Inport
  target_velocity : Inport  Port=2
  1/Voltage : Constant  Value=1/300
  Amps vs time : Scope
      settings: SaveName=ScopeData15
  Constant : Constant  Value=1/0.41
  Product{1..4} (4 alike) : Product  RndMeth=Zero
  Scope{1..5} (5 alike) : Scope
      Scope1 settings: SaveName=ScopeData5
      Scope2 settings: SaveName=ScopeData6
      Scope3 settings: SaveName=ScopeData8
      Scope4 settings: SaveName=ScopeData9
      Scope5 settings: SaveName=ScopeData10
  Sum : Sum  Inputs=|++
  Sum1 : Sum  Inputs=|-+-
  Tractive power vs time : Scope
      settings: SaveName=ScopeData14
  Weight constant : Constant  Value=0.01*weight_N
  WtoKW : Gain  Gain=1/1000
  m_s to mph1 : Gain  Gain=2.24
  multiplication  factor : Gain  Gain=0.0001*weight_N
  multiplication factor : Gain  Gain=0.5*Cd*density*area_sq_m
  multiplication factor1 : Gain  Gain=9.81/16000
  tractive force vs time : Scope
      settings: SaveName=ScopeData13
  Out2 : Outport
  wires:
  Weight constant/1 -> Sum/1
  multiplication  factor/1 -> Sum/2
  Sum/1 -> [roll_resistance], Scope4/1
  [vel_mph] -> multiplication  factor/1
  multiplication factor/1 -> Product1/1
  [vel_m_s] -> multiplication factor/1, Product1/2
  Product1/1 -> [Drag], Scope5/1
  [Torque_request] -> Product2/1
  Constant/1 -> Product2/2
  Product2/1 -> [tractive_force], tractive force vs time/1
  [roll_resistance] -> Sum1/1
  [tractive_force] -> Sum1/2
  [Drag] -> Sum1/3
  Sum1/1 -> multiplication factor1/1
  multiplication factor1/1 -> [acceleration], Scope2/1
  Torque_request/1 -> [Torque_request], Scope1/1
  target_velocity/1 -> m_s to mph1/1, [vel_m_s], Scope3/1
  m_s to mph1/1 -> [vel_mph]
  [acceleration] -> Out2/1
  [tractive_force] -> Product3/1
  [vel_m_s] -> Product3/2
  Product3/1 -> Product4/2, WtoKW/1
  1/Voltage/1 -> Product4/1
  Product4/1 -> Amps vs time/1
  WtoKW/1 -> Tractive power vs time/1

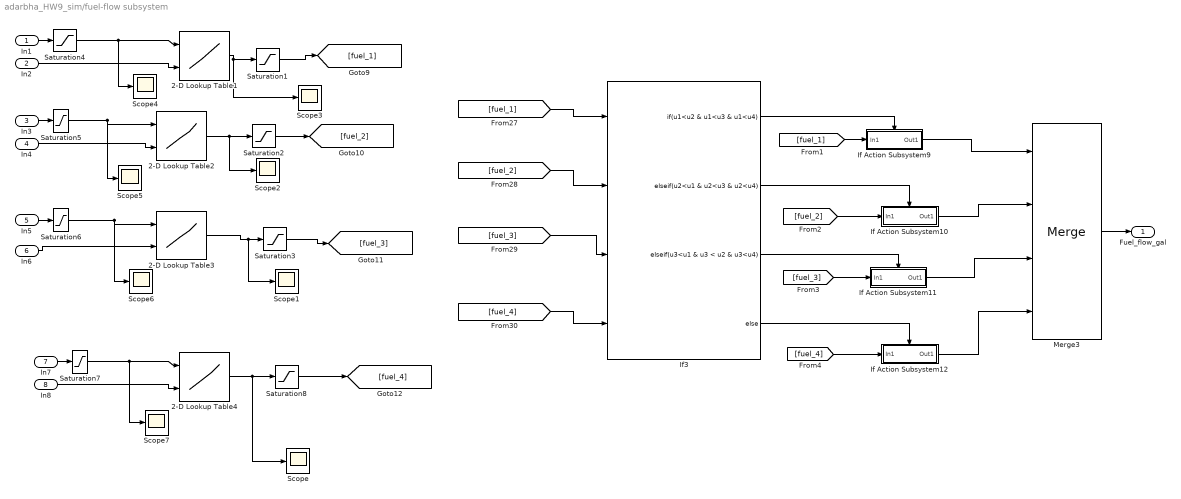
== system adarbha_HW9_sim/fuel-flow subsystem ==
  In1 : Inport
  In2 : Inport  Port=2
  In3 : Inport  Port=3
  In4 : Inport  Port=4
  In5 : Inport  Port=5
  In6 : Inport  Port=6
  In7 : Inport  Port=7
  In8 : Inport  Port=8
  2-D Lookup Table{1..4} (4 alike) : Lookup_n-D  BreakpointsForDimension1=OMEGA_ICE  BreakpointsForDimension2=TORQUE_ICE  Table=FUEL_FLOW  RndMeth=Simplest  InputSameDT=on
  If Action Subsystem10 : Subsystem  TreatAsAtomicUnit=on
  If Action Subsystem11 : Subsystem  TreatAsAtomicUnit=on
  If Action Subsystem12 : Subsystem  TreatAsAtomicUnit=on
  If Action Subsystem9 : Subsystem  TreatAsAtomicUnit=on
  If3 : If  NumInputs=4  IfExpression=u1<u2 & u1<u3 & u1<u4  ElseIfExpressions=u2<u1 & u2<u3 & u2<u4, u3<u1 & u3 < u2 & u3<u4
  Merge3 : Merge  Inputs=4
  Saturation{1..3,8} (4 alike) : Saturate  UpperLimit=Inf  LowerLimit=0.03
  Saturation{4..7} (4 alike) : Saturate  UpperLimit=Inf  LowerLimit=1000
  Scope{,1..7} (8 alike) : Scope
      Scope settings: SaveName=ScopeData47
      Scope1 settings: SaveName=ScopeData50
      Scope2 settings: SaveName=ScopeData51
      Scope3 settings: SaveName=ScopeData52
      Scope4 settings: SaveName=ScopeData55
      Scope5 settings: SaveName=ScopeData56
      Scope6 settings: SaveName=ScopeData57
      Scope7 settings: SaveName=ScopeData58
  Fuel_flow_gal : Outport
  wires:
  2-D Lookup Table1/1 -> Scope3/1, Saturation1/1
  2-D Lookup Table2/1 -> Scope2/1, Saturation2/1
  2-D Lookup Table3/1 -> Scope1/1, Saturation3/1
  [fuel_1] -> If3/1
  [fuel_2] -> If3/2
  [fuel_3] -> If3/3
  [fuel_4] -> If3/4
  If3/1 -> If Action Subsystem9/Action
  If3/2 -> If Action Subsystem10/Action
  [fuel_2] -> If Action Subsystem10/1(In1)
  [fuel_3] -> If Action Subsystem11/1(In1)
  If3/4 -> If Action Subsystem12/Action
  If3/3 -> If Action Subsystem11/Action
  If Action Subsystem9/1(Out1) -> Merge3/1
  If Action Subsystem10/1(Out1) -> Merge3/2
  If Action Subsystem11/1(Out1) -> Merge3/3
  If Action Subsystem12/1(Out1) -> Merge3/4
  In1/1 -> Saturation4/1
  In2/1 -> 2-D Lookup Table1/2
  In3/1 -> Saturation5/1
  In4/1 -> 2-D Lookup Table2/2
  In5/1 -> Saturation6/1
  Merge3/1 -> Fuel_flow_gal/1
  In6/1 -> 2-D Lookup Table3/2
  In7/1 -> Saturation7/1
  In8/1 -> 2-D Lookup Table4/2
  [fuel_1] -> If Action Subsystem9/1(In1)
  [fuel_4] -> If Action Subsystem12/1(In1)
  Saturation4/1 -> 2-D Lookup Table1/1, Scope4/1
  Saturation5/1 -> 2-D Lookup Table2/1, Scope5/1
  2-D Lookup Table4/1 -> Scope/1, Saturation8/1
  Saturation6/1 -> 2-D Lookup Table3/1, Scope6/1
  Saturation7/1 -> 2-D Lookup Table4/1, Scope7/1
  Saturation1/1 -> [fuel_1]
  Saturation2/1 -> [fuel_2]
  Saturation3/1 -> [fuel_3]
  Saturation8/1 -> [fuel_4]

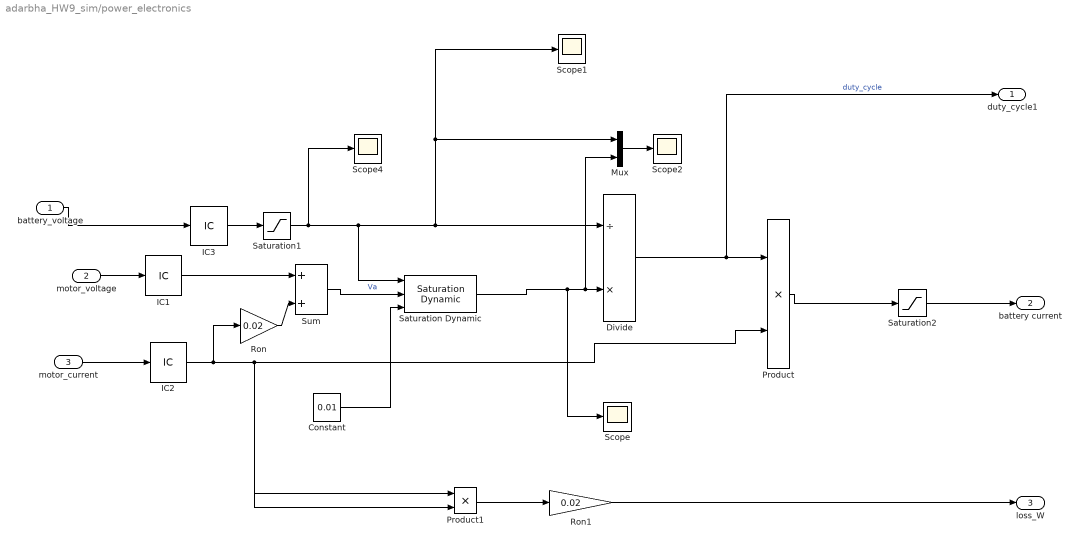
== system adarbha_HW9_sim/power_electronics ==
  battery_voltage : Inport
  motor_voltage : Inport  Port=2
  motor_current : Inport  Port=3
  Constant : Constant  Value=0.01
  Divide : Product  Inputs=/*
  IC1 : InitialCondition  Value=0.01
  IC2 : InitialCondition  Value=0.01
  IC3 : InitialCondition
  Mux : Mux  Inputs=2
  Product : Product  RndMeth=Zero
  Product1 : Product  RndMeth=Zero
  Ron : Gain  Gain=0.02
  Ron1 : Gain  Gain=0.02
  Saturation Dynamic : simulink/Discontinuities/Saturation Dynamic  SystemSampleTime=-1  OutMin=[]  OutMax=[]  OutDataTypeStr=Inherit: Same as second input  OutDataType=fixdt(1, 16)  OutScaling=2^-10  DoSatur=off
  Saturation1 : Saturate  UpperLimit=300  LowerLimit=1  ZeroCross=off
  Saturation2 : Saturate  UpperLimit=Inf  LowerLimit=-100  ZeroCross=off
  Scope{,1..2,4} (4 alike) : Scope
      Scope1 settings: SaveName=ScopeData2
      Scope2 settings: SaveName=ScopeData27
      Scope4 settings: SaveName=ScopeData35
  Sum : Sum  Inputs=|++
  duty_cycle1 : Outport
  battery current : Outport  Port=2
  loss_W : Outport  Port=3
  wires:
  battery_voltage/1 -> IC3/1
  motor_voltage/1 -> IC1/1
  motor_current/1 -> IC2/1
  Divide/1 -> Product/1, duty_cycle1/1  "duty_cycle"
  Product1/1 -> Ron1/1
  Product/1 -> Saturation2/1
  Ron1/1 -> loss_W/1
  Ron/1 -> Sum/2
  IC1/1 -> Sum/1
  IC2/1 -> Product/2, Product1/1, Product1/2, Ron/1
  Saturation2/1 -> battery current/1
  Mux/1 -> Scope2/1
  IC3/1 -> Saturation1/1
  Saturation1/1 -> Scope4/1, Divide/1, Scope1/1, Mux/1, Saturation Dynamic/1
  Saturation Dynamic/1 -> Scope/1, Divide/2, Mux/2
  Sum/1 -> Saturation Dynamic/2  "Va"
  Constant/1 -> Saturation Dynamic/3

== system adarbha_HW9_sim/Gear-look up/If Action Subsystem10 ==
  In1 : Inport
  Action Port : ActionPort  ActionType=elseif
  Out1 : Outport
  wires:
  In1/1 -> Out1/1

== system adarbha_HW9_sim/Gear-look up/If Action Subsystem11 ==
  In1 : Inport
  Action Port : ActionPort  ActionType=elseif
  Out1 : Outport
  wires:
  In1/1 -> Out1/1

== system adarbha_HW9_sim/Gear-look up/If Action Subsystem12 ==
  In1 : Inport
  Action Port : ActionPort  ActionType=else
  Out1 : Outport
  wires:
  In1/1 -> Out1/1

== system adarbha_HW9_sim/Gear-look up/If Action Subsystem9 ==
  In1 : Inport
  Action Port : ActionPort  ActionType=then
  Out1 : Outport
  wires:
  In1/1 -> Out1/1

== system adarbha_HW9_sim/If Action Subsystem1/If Action Subsystem ==
  In1 : Inport
  Action Port : ActionPort  ActionType=then
  Out1 : Outport
  wires:
  In1/1 -> Out1/1

== system adarbha_HW9_sim/If Action Subsystem1/If Action Subsystem1 ==
  In1 : Inport
  Action Port : ActionPort  ActionType=elseif
  Out1 : Outport
  wires:
  In1/1 -> Out1/1

== system adarbha_HW9_sim/If Action Subsystem1/If Action Subsystem2 ==
  In1 : Inport
  Action Port : ActionPort  ActionType=elseif
  Out1 : Outport
  wires:
  In1/1 -> Out1/1

== system adarbha_HW9_sim/If Action Subsystem1/If Action Subsystem3 ==
  In1 : Inport
  Action Port : ActionPort  ActionType=else
  Out1 : Outport
  wires:
  In1/1 -> Out1/1

== system adarbha_HW9_sim/fuel-flow subsystem/If Action Subsystem10 ==
  In1 : Inport
  Action Port : ActionPort  ActionType=elseif
  Out1 : Outport
  wires:
  In1/1 -> Out1/1

== system adarbha_HW9_sim/fuel-flow subsystem/If Action Subsystem11 ==
  In1 : Inport
  Action Port : ActionPort  ActionType=elseif
  Out1 : Outport
  wires:
  In1/1 -> Out1/1

== system adarbha_HW9_sim/fuel-flow subsystem/If Action Subsystem12 ==
  In1 : Inport
  Action Port : ActionPort  ActionType=else
  Out1 : Outport
  wires:
  In1/1 -> Out1/1

== system adarbha_HW9_sim/fuel-flow subsystem/If Action Subsystem9 ==
  In1 : Inport
  Action Port : ActionPort  ActionType=then
  Out1 : Outport
  wires:
  In1/1 -> Out1/1
